simulink model "P1C2"  (R2023b)
settings: Solver=VariableStepAuto  StartTime=0.0  StopTime=75  RelTol=1e-3
settings Model: Creator=tanvi  LastModifiedBy=tanvi

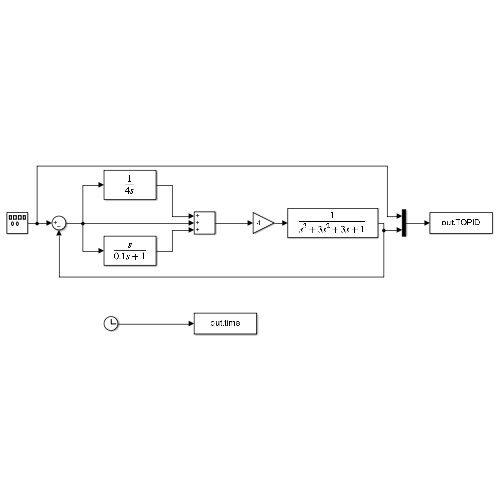
[thumbnail: Simulink's stored preview of the top-level diagram]
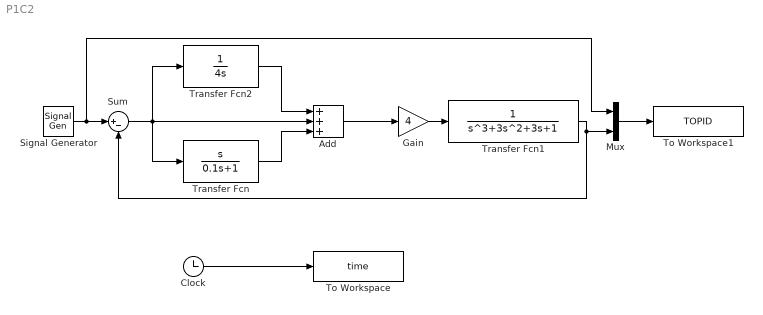
== system P1C2 ==
  Add : Sum  Inputs=+++
  Clock : Clock
  Gain : Gain  Gain=4
  Mux : Mux  Inputs=2
  Signal Generator : SignalGenerator  WaveForm=square  Frequency=0.02
  Sum : Sum  Inputs=|+-
  To Workspace : ToWorkspace  VariableName=time  SampleTime=-1
  To Workspace1 : ToWorkspace  VariableName=TOPID  SampleTime=-1
  Transfer Fcn : TransferFcn  Numerator=[1 0]  Denominator=[0.1 1]
  Transfer Fcn1 : TransferFcn  Denominator=[1 3 3 1]
  Transfer Fcn2 : TransferFcn  Denominator=[4 0]
  wires:
  Add/1 -> Gain/1
  Mux/1 -> To Workspace1/1
  Transfer Fcn/1 -> Add/3
  Signal Generator/1 -> Mux/1, Sum/1
  Transfer Fcn1/1 -> Sum/2, Mux/2
  Clock/1 -> To Workspace/1
  Sum/1 -> Transfer Fcn/1, Add/2, Transfer Fcn2/1
  Gain/1 -> Transfer Fcn1/1
  Transfer Fcn2/1 -> Add/1
